simulink model "invertedPendulum"  (R2016a)
settings: Solver=VariableStepAuto  StartTime=0.0  StopTime=10  MaxStep=1e-3  MinStep=1e-6  RelTol=1e-5  AbsTol=1e-5
values from neighbouring files (symbols this model uses):
  beta = 0.001    [parameters.mat]
  f_sampling = 30    [parameters.mat]
  g = 9.80665    [parameters.mat]
  l = 0.0825    [parameters.mat]
  m = 0.784    [parameters.mat]
  r = 0.0325    [parameters.mat]
libraries: simulink x1
settings Model: Creator=hda8rt  LastModifiedBy=Adina Haendel
settings SolverCC: InitialStep=1e-4
settings DataIOCC: LimitDataPoints=on
settings DebuggingCC: AllowSymbolicDim=off
settings ModelReferenceCC: PropagateSignalLabelsOutOfModel=off
settings GRTTargetCC: GeneratePreprocessorConditionals=Use local settings

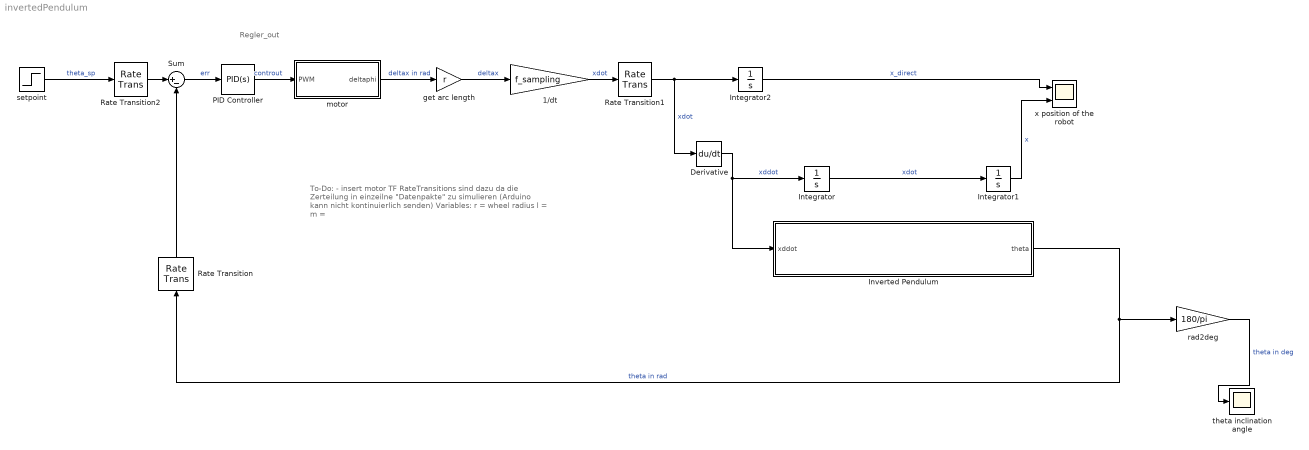
== system invertedPendulum ==
  note: Regler_out
  note: To-Do:
      | - insert motor TF
      |
      |
      |
      | RateTransitions sind dazu da die Zerteilung
      | in einzeilne "Datenpakte" zu simulieren
      | (Arduino kann nicht kontinuierlich senden)
      |
      | Variables:
      | r = wheel radius
      | l =
      | m =
  1/dt : Gain  Gain=f_sampling
  Derivative : Derivative
  Integrator : Integrator
  Integrator1 : Integrator
  Integrator2 : Integrator
  Inverted Pendulum : Subsystem
  PID Controller : simulink/Continuous/PID Controller  Controller=PID  TimeDomain=Continuous-time  SampleTime=-1  IntegratorMethod=Forward Euler  FilterMethod=Forward Euler  Form=Parallel  UseFilter=on  ControllerParametersSource=internal  P=1  I=1  D=0  N=100  InitialConditionSource=internal  InitialConditionForIntegrator=0  InitialConditionForFilter=0  ExternalReset=none  LimitOutput=off  UpperSaturationLimit=inf  LowerSaturationLimit=-inf  LinearizeAsGain=on  AntiWindupMode=none  Kb=1  TrackingMode=off  Kt=1  PParamMin=[]  PParamMax=[]  IParamMin=[]  IParamMax=[]  DParamMin=[]  DParamMax=[]  NParamMin=[]  NParamMax=[]  KbParamMin=[]  KbParamMax=[]  KtParamMin=[]  KtParamMax=[]  POutMin=[]  POutMax=[]  IOutMin=[]  IOutMax=[]  DOutMin=[]  DOutMax=[]  NOutMin=[]  NOutMax=[]  KbOutMin=[]  KbOutMax=[]  KtOutMin=[]  KtOutMax=[]  IntegratorOutMin=[]  IntegratorOutMax=[]  FilterOutMin=[]  FilterOutMax=[]  SumOutMin=[]  SumOutMax=[]  SumI1OutMin=[]  SumI1OutMax=[]  SumI2OutMin=[]  SumI2OutMax=[]  SumI3OutMin=[]  SumI3OutMax=[]  SumDOutMin=[]  SumDOutMax=[]  SaturationOutMin=[]  SaturationOutMax=[]  IntegratorContinuousStateAttributes=''  IntegratorStateMustResolveToSignalObject=off  IntegratorRTWStateStorageClass=Auto  FilterContinuousStateAttributes=''  FilterStateMustResolveToSignalObject=off  FilterRTWStateStorageClass=Auto  DifferentiatorICPrevScaledInput=0  DifferentiatorOutMin=[]  DifferentiatorOutMax=[]
  Rate Transition : RateTransition  OutPortSampleTime=1/f_sampling
  Rate Transition1 : RateTransition  OutPortSampleTimeOpt=Inherit  OutPortSampleTime=1/f_sampling
  Rate Transition2 : RateTransition  OutPortSampleTime=1/f_sampling
  Sum : Sum  Inputs=|+-
  get arc length : Gain  Gain=r
  motor : Subsystem
  rad2deg : Gain  Gain=180/pi
  setpoint : Step  Time=20  After=0*pi/180  SampleTime=0
  theta inclination angle : Scope
  x position of the robot : Scope  NumInputPorts=2
  wires:
  Integrator/1 -> Integrator1/1  "xdot"
  Integrator1/1 -> x position of the robot/2  "x"
  rad2deg/1 -> theta inclination angle/1  "theta in deg"
  Inverted Pendulum/1(theta) -> rad2deg/1, Rate Transition/1  "theta in rad"
  setpoint/1 -> Rate Transition2/1  "theta_sp"
  Rate Transition/1 -> Sum/2
  Rate Transition2/1 -> Sum/1
  Sum/1 -> PID Controller/1  "err"
  get arc length/1 -> 1/dt/1  "deltax"
  PID Controller/1 -> motor/1(PWM)  "controut"
  1/dt/1 -> Rate Transition1/1  "xdot"
  Rate Transition1/1 -> Integrator2/1, Derivative/1  "xdot"
  Derivative/1 -> Integrator/1, Inverted Pendulum/1(xddot)  "xddot"
  Integrator2/1 -> x position of the robot/1  "x_direct"
  motor/1(deltaphi) -> get arc length/1  "deltax in rad"

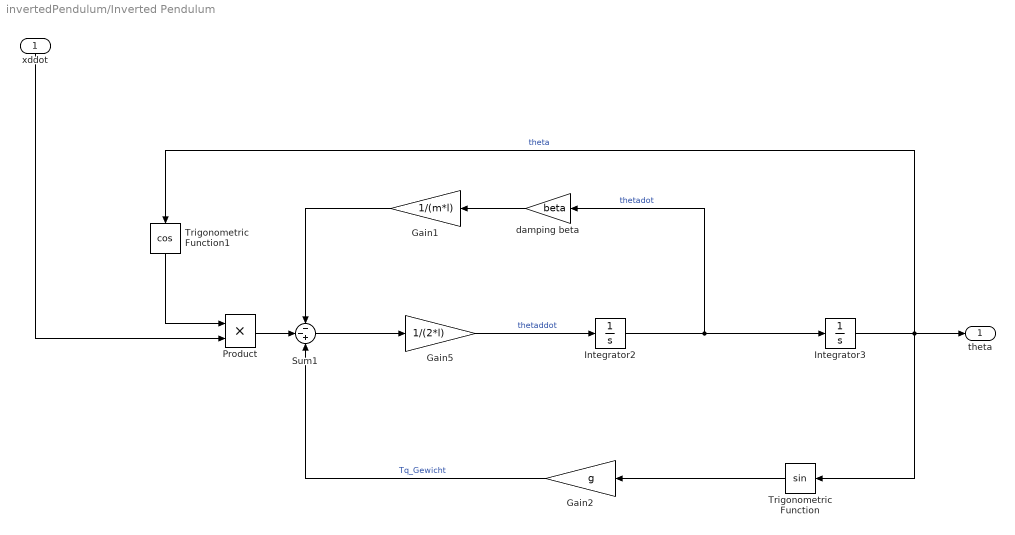
== system invertedPendulum/Inverted Pendulum ==
  xddot : Inport
  Gain1 : Gain  Gain=1/(m*l)
  Gain2 : Gain  Gain=g
  Gain5 : Gain  Gain=1/(2*l)
  Integrator2 : Integrator
  Integrator3 : Integrator  InitialCondition=0*pi/180
  Product : Product  Inputs=**
  Sum1 : Sum  Inputs=--+
  Trigonometric Function : Trigonometry
  Trigonometric Function1 : Trigonometry  Operator=cos
  damping beta : Gain  Gain=beta
  theta : Outport
  wires:
  Integrator3/1 -> Trigonometric Function1/1, Trigonometric Function/1, theta/1  "theta"
  Gain5/1 -> Integrator2/1  "thetaddot"
  Sum1/1 -> Gain5/1
  Integrator2/1 -> Integrator3/1, damping beta/1  "thetadot"
  xddot/1 -> Product/2
  damping beta/1 -> Gain1/1
  Gain2/1 -> Sum1/3  "Tq_Gewicht"
  Gain1/1 -> Sum1/1
  Trigonometric Function/1 -> Gain2/1
  Trigonometric Function1/1 -> Product/1
  Product/1 -> Sum1/2

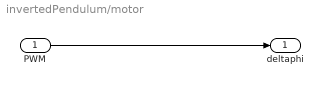
== system invertedPendulum/motor ==
  PWM : Inport
  deltaphi : Outport
  wires:
  PWM/1 -> deltaphi/1
